simulink library "se2a_controller_lib"  (R2018b)
settings: Solver=VariableStepAuto  StartTime=0.0  StopTime=10.0  RelTol=1e-3
undefined symbols (not defined in the file or in its folder): aircraft, DiscIntNeverNeededParam, gla_indi, pitch_rate_controller
libraries: filters_lib x12, ca_lib x2, simulink x1
settings Model: Creator=Ybeyer  LastModifiedBy=yannic
settings SFSimCC: SimUseLocalCustomCode=off
settings RTWCC: RTWUseLocalCustomCode=off
settings CodeAppCC: StateflowObjectComments=on

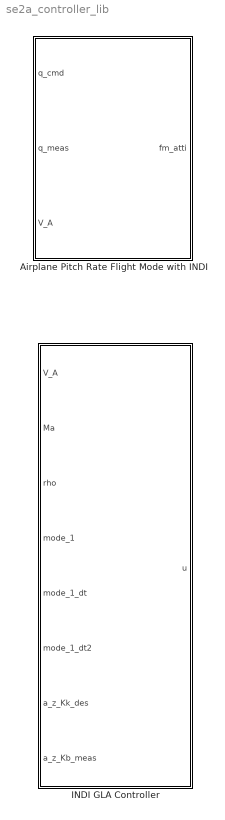
== system se2a_controller_lib ==
  Airplane Pitch Rate Flight Mode with INDI : Subsystem  mask{fm=pitch_rate_controller}
      mask prompts: fm "Pitch rate controller parameters struct"
      mask DialogControl DescGroupVar Prompt: Airplane Pitch Rate Controller with INDI
  INDI GLA Controller : Subsystem  mask{gla_indi=gla_indi}
      mask prompts: gla_indi "Controller parameters struct"
      mask init:
      | % to be controlled mode numbers (non-tunable parameter)
      | mcidx = gla_indi.mcidx;
      mask DialogControl DescGroupVar Prompt: INDI GLA Controller

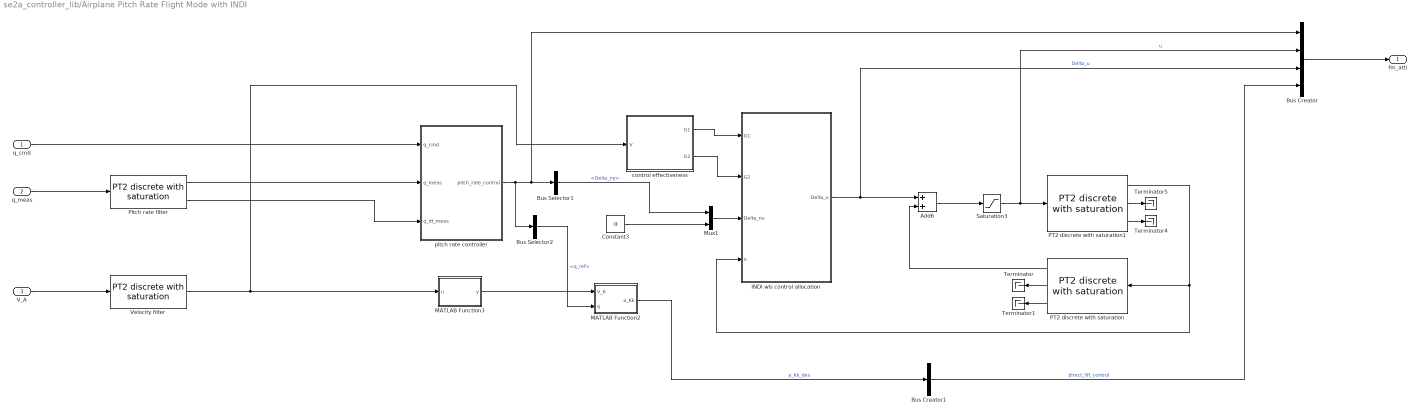
== system se2a_controller_lib/Airplane Pitch Rate Flight Mode with INDI ==
  q_cmd : Inport  SampleTime=fm.sample_time
  q_meas : Inport  Port=2  SampleTime=fm.sample_time
  V_A : Inport  Port=3  SampleTime=fm.sample_time
  Add6 : Sum
  Bus Creator : BusCreator  Inputs=4
  Bus Creator1 : BusCreator  Inputs=1
  Bus Selector1 : BusSelector  OutputSignals=pseudo_control.Delta_ny
  Bus Selector2 : BusSelector  OutputSignals=reference.q_ref
  Constant3 : Constant  Value=0
  INDI wls control allocation : Subsystem  mask{ca=fm.ca, is_Delta_W_v_check=off, is_W_check=off, is_iter_check=off}
      mask prompts: ca "control allocation parameters struct"; is_Delta_W_v_check "enable online adjustment of diag W_v"; is_W_check "enable output "optimal active set" W"; is_iter_check "enable output "number of iterations" iter"
      mask init:
      | caIndiWlsHlcBlockInit(is_Delta_W_v_check,is_W_check,is_iter_check)
      mask DialogControl DescGroupVar Prompt: INDI high level control allocation
      mask DialogControl DescTextVar Prompt: It wraps the INDI control allocation block and adds some high level usability features.
      mask DialogControl Control2 Prompt: This block makes manual throttle control possible. Moreover, it not only considers the control effectiveness G1 but also the effectiveness of the control input derivative G2 [1].
      mask DialogControl Control3 Prompt: [1] Smeur, E. J., Chu, Q., & de Croon, G. C. (2016). Adaptive incremental nonlinear dynamic inversion for attitude control of micro air vehicles. Journal of Guidance, Control, and Dynamics, 39(3), 450-461.
      mask DialogControl Control4 Prompt: To load a control allocation parameters struct, see controlAllocationWlsLoadParams
  MATLAB Function2 : MATLAB Function  TreatAsAtomicUnit=on
  MATLAB Function3 : MATLAB Function  TreatAsAtomicUnit=on
  Mux1 : Mux  Inputs=2
  PT2 discrete with saturation : filters_lib/PT2 discrete with saturation  param_src=internal  omega=fm.sflt.omega  d=fm.sflt.D  x_dt2_max=inf  x_dt2_min=-inf  x_dt_max=inf  x_dt_min=-inf  x_max=inf  x_min=-inf  y_0_src=internal  x_init=0  y_dt_0_src=internal  x_dt_init=0  is_y_dt_checked=on  is_y_dt2_checked=on
      settings: SourceProductName=LADAC
  PT2 discrete with saturation1 : filters_lib/PT2 discrete with saturation  param_src=internal  omega=fm.servo.omega  d=fm.servo.D  x_dt2_max=inf  x_dt2_min=-inf  x_dt_max=inf  x_dt_min=-inf  x_max=inf  x_min=-inf  y_0_src=internal  x_init=0  y_dt_0_src=internal  x_dt_init=0  is_y_dt_checked=on  is_y_dt2_checked=on
      settings: SourceProductName=LADAC
  Pitch rate filter : filters_lib/PT2 discrete with saturation  param_src=internal  omega=fm.sflt.omega  d=fm.sflt.D  x_dt2_max=inf  x_dt2_min=-inf  x_dt_max=inf  x_dt_min=-inf  x_max=inf  x_min=-inf  y_0_src=internal  x_init=0  y_dt_0_src=internal  x_dt_init=0  is_y_dt_checked=on  is_y_dt2_checked=off
      settings: SourceProductName=LADAC
  Saturation3 : Saturate  UpperLimit=fm.ca.u_max  LowerLimit=fm.ca.u_min
  Terminator{,1,4..5} (4 alike) : Terminator
  Velocity filter : filters_lib/PT2 discrete with saturation  param_src=internal  omega=fm.sflt.omega  d=fm.sflt.D  x_dt2_max=inf  x_dt2_min=-inf  x_dt_max=inf  x_dt_min=-inf  x_max=inf  x_min=-inf  y_0_src=internal  x_init=0  y_dt_0_src=internal  x_dt_init=0  is_y_dt_checked=off  is_y_dt2_checked=off
      settings: SourceProductName=LADAC
  control effectiveness : Subsystem
  pitch rate controller : Subsystem
  fm_atti : Outport  SampleTime=fm.sample_time
  wires:
  Constant3/1 -> Mux1/2
  Mux1/1 -> INDI wls control allocation/3(Delta_nu)
  Bus Selector2/1 -> MATLAB Function2/2(q)  "<q_ref>"
  MATLAB Function2/1(a_Kk) -> Bus Creator1/1  "a_Kk_des"
  MATLAB Function3/1(y) -> MATLAB Function2/1(V_K)
  Bus Creator1/1 -> Bus Creator/4  "direct_lift_control"
  Velocity filter/1 -> control effectiveness/1(V), MATLAB Function3/1(u)
  pitch rate controller/1(pitch_rate_control) -> Bus Selector1/1, Bus Creator/1, Bus Selector2/1
  Pitch rate filter/1 -> pitch rate controller/2(q_meas)
  q_cmd/1 -> pitch rate controller/1(q_cmd)
  Saturation3/1 -> Bus Creator/2, PT2 discrete with saturation1/1  "u"
  Bus Selector1/1 -> Mux1/1  "<Delta_ny>"
  PT2 discrete with saturation1/1 -> PT2 discrete with saturation/1, INDI wls control allocation/4(u)
  control effectiveness/2(G2) -> INDI wls control allocation/2(G2)
  Add6/1 -> Saturation3/1
  control effectiveness/1(G1) -> INDI wls control allocation/1(G1)
  INDI wls control allocation/1(Delta_u) -> Add6/1, Bus Creator/3  "Delta_u"
  PT2 discrete with saturation/2 -> Terminator/1
  PT2 discrete with saturation/3 -> Terminator1/1
  Bus Creator/1 -> fm_atti/1
  PT2 discrete with saturation/1 -> Add6/2
  PT2 discrete with saturation1/3 -> Terminator4/1
  PT2 discrete with saturation1/2 -> Terminator5/1
  q_meas/1 -> Pitch rate filter/1
  Pitch rate filter/2 -> pitch rate controller/3(q_dt_meas)
  V_A/1 -> Velocity filter/1

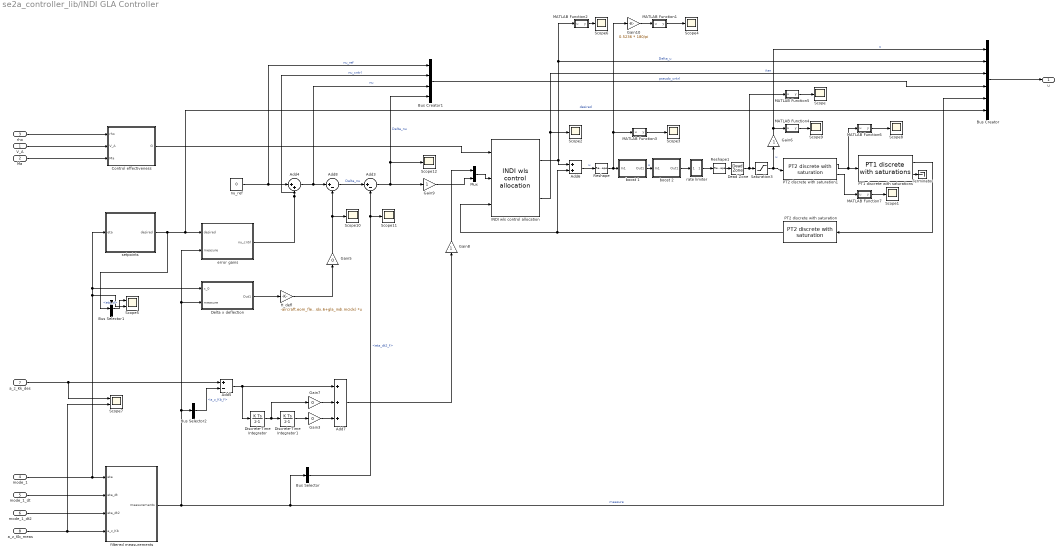
== system se2a_controller_lib/INDI GLA Controller ==
  V_A : Inport  SampleTime=gla_indi.ts
  Ma : Inport  Port=2  SampleTime=gla_indi.ts
  rho : Inport  Port=3  SampleTime=gla_indi.ts
  mode_1 : Inport  Port=4  SampleTime=gla_indi.ts
  mode_1_dt : Inport  Port=5  SampleTime=gla_indi.ts
  mode_1_dt2 : Inport  Port=6  SampleTime=gla_indi.ts
  a_z_Kk_des : Inport  Port=7  SampleTime=gla_indi.ts
  a_z_Kb_meas : Inport  Port=8  SampleTime=gla_indi.ts
  Add3 : Sum  Inputs=|+-
  Add4 : Sum  Inputs=|++
  Add5 : Sum  Inputs=+-
  Add6 : Sum
  Add7 : Sum  Inputs=+++
  Add8 : Sum  Inputs=|+-
  Bus Creator : BusCreator  Inputs=6
  Bus Creator1 : BusCreator  Inputs=4
  Bus Selector : BusSelector  OutputSignals=eta_dt2_f
  Bus Selector1 : BusSelector  OutputSignals=eta_d
  Bus Selector2 : BusSelector  OutputSignals=a_z_Kb_f
  Control effectiveness : Subsystem  mask{cel=gla_indi.ce}
      mask prompts: cel "Control effectiveness parameters struct"
      mask DialogControl DescGroupVar Prompt: Control effectiveness of LADs
  Dead Zone : DeadZone  LowerValue=-gla_indi.udead  UpperValue=gla_indi.udead  SaturateOnIntegerOverflow=on
  Delta x deflection : Subsystem
  Discrete-Time Integrator : DiscreteIntegrator  SampleTime=-1  ICPrevOutput=DiscIntNeverNeededParam  ICPrevScaledInput=DiscIntNeverNeededParam
  Discrete-Time Integrator1 : DiscreteIntegrator  SampleTime=-1  ICPrevOutput=DiscIntNeverNeededParam  ICPrevScaledInput=DiscIntNeverNeededParam
  Gain10 : Gain  Gain=0.5236 * 180/pi
  Gain3 : Gain  Gain=0
  Gain5 : Gain  Gain=0
  Gain6 : Gain
  Gain7 : Gain  Gain=0
  Gain8 : Gain
  Gain9 : Gain
  H_defl : Gain  Gain=-aircraft.eom_flexible.structure_red.M_inv(6+gla_indi.mcidx,6+gla_indi.mcidx)*aircraft.eom_flexible.structure_red.K(6+gla_indi.mcidx,6+gla_indi.mcidx)  Multiplication=Matrix(K*u)
  INDI wls control allocation : ca_lib/INDI wls control allocation  ca=gla_indi.ca  is_Delta_u_d_checked=off  is_Delta_gamma_checked=off  is_Delta_W_v_checked=off  is_Delta_u_max_checked=off  is_W_checked=off  is_iter_checked=on
      settings: SourceProductName=LADAC
  MATLAB Function1 : MATLAB Function  TreatAsAtomicUnit=on
  MATLAB Function2 : MATLAB Function  TreatAsAtomicUnit=on
  MATLAB Function3 : MATLAB Function  TreatAsAtomicUnit=on
  MATLAB Function4 : MATLAB Function  TreatAsAtomicUnit=on
  MATLAB Function5 : MATLAB Function  TreatAsAtomicUnit=on
  MATLAB Function6 : MATLAB Function  TreatAsAtomicUnit=on
  MATLAB Function7 : MATLAB Function  TreatAsAtomicUnit=on
  Mux : Mux  Inputs=2
  PT1 discrete with saturations : filters_lib/PT1 discrete with saturations  T=gla_indi.atc  x_max=inf  x_min=-inf  x_dt_max=inf  x_dt_min=-inf  x_init=0
      settings: SourceProductName=LADAC
  PT2 discrete with saturation : filters_lib/PT2 discrete with saturation  param_src=internal  omega=gla_indi.sflt.omega  d=gla_indi.sflt.d  x_dt2_max=inf  x_dt2_min=-inf  x_dt_max=inf  x_dt_min=-inf  x_max=inf  x_min=-inf  y_0_src=internal  x_init=0  y_dt_0_src=internal  x_dt_init=0  is_y_dt_checked=off  is_y_dt2_checked=off
      settings: SourceProductName=LADAC
  PT2 discrete with saturation1 : filters_lib/PT2 discrete with saturation  param_src=internal  omega=2/gla_indi.dtc  d=1  x_dt2_max=inf  x_dt2_min=-inf  x_dt_max=aircraft.actuators.LAD.defl_rate_max/aircraft.actuators.LAD.defl_max  x_dt_min=aircraft.actuators.LAD.defl_rate_min/aircraft.actuators.LAD.defl_max  x_max=inf  x_min=-inf  y_0_src=internal  x_init=0  y_dt_0_src=internal  x_dt_init=0  is_y_dt_checked=on  is_y_dt2_checked=off
      settings: SourceProductName=LADAC
  Reshape : Reshape  OutputDimensionality=Row vector (2-D)
  Reshape1 : Reshape
  Saturation3 : Saturate  UpperLimit=gla_indi.ca.u_max  LowerLimit=gla_indi.ca.u_min
  Scope{,1..4,6,8..12} (11 alike) : Scope
  Scope5 : Scope  NumInputPorts=2
  Scope7 : Scope  NumInputPorts=2
  Terminator : Terminator
  boost 1 : Subsystem
  boost 2 : Subsystem
  error gains : Subsystem
  filtered measurements : Subsystem
  nu_ref : Constant  Value=0
  rate limiter : Subsystem
  setpoints : Subsystem
  u : Outport
  wires:
  Add4/1 -> Bus Creator1/3, Add8/1  "nu"
  Add8/1 -> Add3/1  "Delta_nu"
  nu_ref/1 -> Add4/1, Bus Creator1/1  "nu_ref"
  filtered measurements/1(measurements) -> Bus Creator/5, Bus Selector/1, Bus Selector2/1, error gains/2(measure), Delta x deflection/2(measure)  "measure"
  INDI wls control allocation/1 -> Add6/1, MATLAB Function2/1(u), Bus Creator/2  "Delta_u"
  Saturation3/1 -> PT2 discrete with saturation1/1, Gain6/1  "u"
  PT1 discrete with saturations/1 -> PT2 discrete with saturation/1
  INDI wls control allocation/2 -> Bus Creator/3, Scope2/1  "iter"
  Dead Zone/1 -> MATLAB Function5/1(u), Saturation3/1
  mode_1_dt/1 -> filtered measurements/2(eta_dt)
  mode_1_dt2/1 -> filtered measurements/3(eta_dt2)
  Bus Creator/1 -> u/1
  error gains/1(nu_cntrl) -> Bus Creator1/2, Add4/2  "nu_cntrl"
  setpoints/1(desired) -> Bus Selector1/1, error gains/1(desired), Bus Creator/6  "desired"
  Bus Creator1/1 -> Bus Creator/4  "pseudo_cntrl"
  Bus Selector/1 -> Add3/2, Scope11/1  "<eta_dt2_f>"
  Control effectiveness/1(G) -> INDI wls control allocation/1
  rho/1 -> Control effectiveness/1(rho)
  V_A/1 -> Control effectiveness/2(V_A)
  Ma/1 -> Control effectiveness/3(Ma)
  H_defl/1 -> Gain5/1
  Gain5/1 -> Add8/2, Scope10/1
  Gain6/1 -> MATLAB Function4/1(u), Bus Creator/1  "u"
  Reshape1/1 -> Dead Zone/1
  Add6/1 -> Reshape/1  "u"
  Reshape/1 -> Gain10/1, MATLAB Function3/1(u), boost 1/1(In1)
  a_z_Kk_des/1 -> Add5/1, Scope7/1
  a_z_Kb_meas/1 -> Scope7/2, filtered measurements/4(a_z_Kb)
  Mux/1 -> INDI wls control allocation/2
  Add5/1 -> Discrete-Time Integrator/1, Add7/1
  Gain8/1 -> Mux/1
  Gain9/1 -> Mux/2
  PT2 discrete with saturation1/1 -> MATLAB Function6/1(u), PT1 discrete with saturations/1
  PT1 discrete with saturations/2 -> Terminator/1
  boost 1/1(Out1) -> boost 2/1(In1)  "u"
  PT2 discrete with saturation/1 -> Add6/2, INDI wls control allocation/3
  Discrete-Time Integrator/1 -> Gain7/1, Discrete-Time Integrator1/1
  Discrete-Time Integrator1/1 -> Gain3/1
  Add7/1 -> Gain8/1
  Gain3/1 -> Add7/3
  Gain7/1 -> Add7/2
  PT2 discrete with saturation1/2 -> MATLAB Function7/1(u)
  Gain10/1 -> MATLAB Function1/1(u)
  MATLAB Function1/1(y) -> Scope4/1
  MATLAB Function2/1(y) -> Scope6/1
  MATLAB Function3/1(y) -> Scope3/1
  MATLAB Function4/1(y) -> Scope9/1
  MATLAB Function5/1(y) -> Scope/1
  MATLAB Function6/1(y) -> Scope8/1
  MATLAB Function7/1(y) -> Scope1/1
  boost 2/1(Out1) -> rate limiter/1(In1)
  rate limiter/1(Out1) -> Reshape1/1
  Add3/1 -> Gain9/1, Bus Creator1/4, Scope12/1  "Delta_nu"
  Delta x deflection/1(Out1) -> H_defl/1
  Bus Selector1/1 -> Scope5/1  "<eta_d>"
  mode_1/1 -> filtered measurements/1(eta), setpoints/1(eta), Delta x deflection/1(x_0), Scope5/2
  Bus Selector2/1 -> Add5/2  "<a_z_Kb_f>"

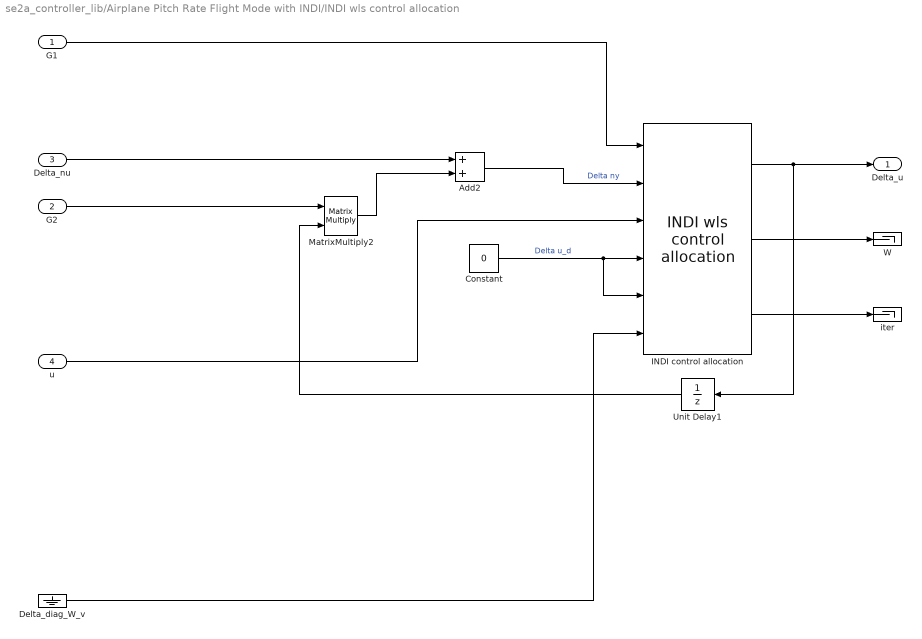
== system se2a_controller_lib/Airplane Pitch Rate Flight Mode with INDI/INDI wls control allocation ==
  G1 : Inport
  G2 : Inport  Port=2
  Delta_nu : Inport  Port=3
  u : Inport  Port=4
  Add2 : Sum
  Constant : Constant  Value=0
  Delta_diag_W_v : Ground
  INDI control allocation : ca_lib/INDI wls control allocation  ca=ca  is_Delta_u_d_checked=on  is_Delta_gamma_checked=on  is_Delta_W_v_checked=on  is_Delta_u_max_checked=off  is_W_checked=on  is_iter_checked=on
      settings: SourceProductName=LADAC
  MatrixMultiply2 : Product  Multiplication=Matrix(*)
  Unit Delay1 : UnitDelay  SampleTime=-1
  W : Terminator
  iter : Terminator
  Delta_u : Outport
  wires:
  G2/1 -> MatrixMultiply2/1
  MatrixMultiply2/1 -> Add2/2
  G1/1 -> INDI control allocation/1
  Add2/1 -> INDI control allocation/2  "Delta ny"
  u/1 -> INDI control allocation/3
  INDI control allocation/1 -> Unit Delay1/1, Delta_u/1
  Delta_nu/1 -> Add2/1
  Unit Delay1/1 -> MatrixMultiply2/2
  Constant/1 -> INDI control allocation/4, INDI control allocation/5  "Delta u_d"
  Delta_diag_W_v/1 -> INDI control allocation/6
  INDI control allocation/3 -> iter/1
  INDI control allocation/2 -> W/1

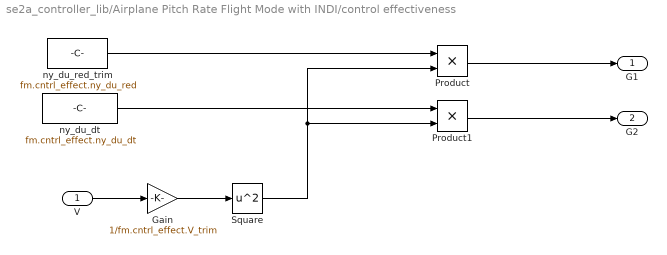
== system se2a_controller_lib/Airplane Pitch Rate Flight Mode with INDI/control effectiveness ==
  V : Inport
  Gain : Gain  Gain=1/fm.cntrl_effect.V_trim
  Product : Product
  Product1 : Product
  Square : Math  Operator=square  SaturateOnIntegerOverflow=on
  ny_du_dt : Constant  Value=fm.cntrl_effect.ny_du_dt
  ny_du_red_trim : Constant  Value=fm.cntrl_effect.ny_du_red
  G1 : Outport
  G2 : Outport  Port=2
  wires:
  ny_du_dt/1 -> Product1/1
  ny_du_red_trim/1 -> Product/1
  V/1 -> Gain/1
  Gain/1 -> Square/1
  Product/1 -> G1/1
  Square/1 -> Product1/2, Product/2
  Product1/1 -> G2/1

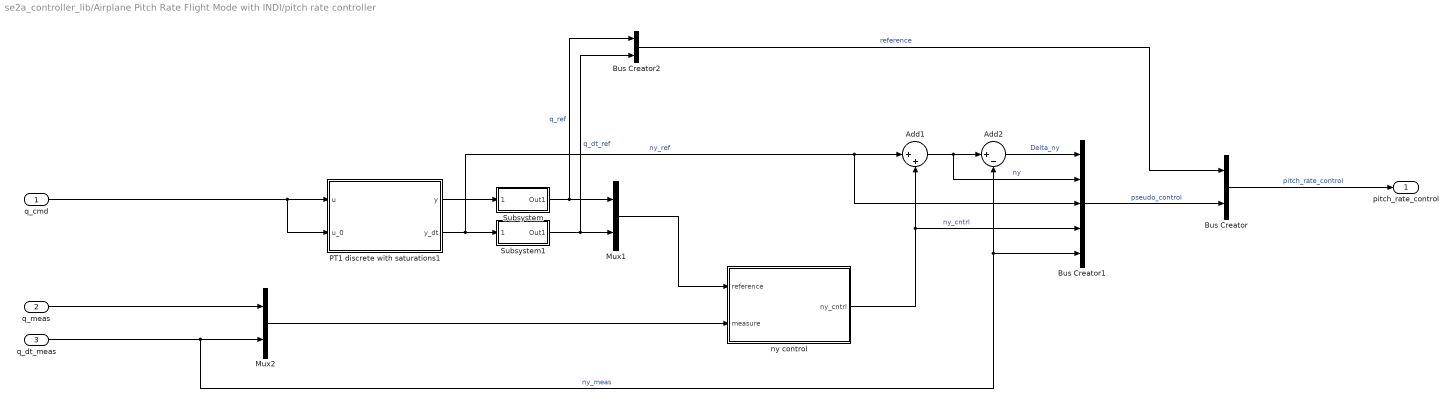
== system se2a_controller_lib/Airplane Pitch Rate Flight Mode with INDI/pitch rate controller ==
  q_cmd : Inport
  q_meas : Inport  Port=2
  q_dt_meas : Inport  Port=3
  Add1 : Sum  Inputs=|++
  Add2 : Sum  Inputs=|+-
  Bus Creator : BusCreator  Inputs=2
  Bus Creator1 : BusCreator  Inputs=5
  Bus Creator2 : BusCreator  Inputs=2
  Mux1 : Mux  Inputs=2
  Mux2 : Mux  Inputs=2
  PT1 discrete with saturations1 : Subsystem  mask{T=fm.rm.T, x_max=inf, x_min=-inf, x_dt_max=inf, x_dt_min=-inf, x_init=0}
      mask prompts: T "Time constant"; x_max "Maximum output"; x_min "Minimum output"; x_dt_max "Maximum output rate"; x_dt_min "Minimum output rate"; x_init "Initial output"
  Subsystem : Subsystem
  Subsystem1 : Subsystem
  ny control : Subsystem
  pitch_rate_control : Outport
  wires:
  Bus Creator2/1 -> Bus Creator/1  "reference"
  Mux2/1 -> ny control/2(measure)
  ny control/1(ny_cntrl) -> Add1/2, Bus Creator1/4  "ny_cntrl"
  q_dt_meas/1 -> Mux2/2, Bus Creator1/5, Add2/2  "ny_meas"
  q_meas/1 -> Mux2/1
  Subsystem1/1(Out1) -> Mux1/2, Bus Creator2/2  "q_dt_ref"
  q_cmd/1 -> PT1 discrete with saturations1/1(u), PT1 discrete with saturations1/2("u_0 ")
  Subsystem/1(Out1) -> Mux1/1, Bus Creator2/1  "q_ref"
  PT1 discrete with saturations1/2(y_dt) -> Add1/1, Bus Creator1/3, Subsystem1/1(<x_ref>)  "ny_ref"
  Add2/1 -> Bus Creator1/1  "Delta_ny"
  Bus Creator/1 -> pitch_rate_control/1  "pitch_rate_control"
  PT1 discrete with saturations1/1(y) -> Subsystem/1(<x_ref>)
  Bus Creator1/1 -> Bus Creator/2  "pseudo_control"
  Add1/1 -> Bus Creator1/2, Add2/1  "ny"
  Mux1/1 -> ny control/1(reference)

== system se2a_controller_lib/INDI GLA Controller/Control effectiveness ==
  rho : Inport
  V_A : Inport  Port=2
  Ma : Inport  Port=3
  Control effectiveness : MATLAB Function  TreatAsAtomicUnit=on
  G : Outport
  wires:
  Ma/1 -> Control effectiveness/3(Ma)
  rho/1 -> Control effectiveness/1(rho)
  Control effectiveness/1(G) -> G/1
  V_A/1 -> Control effectiveness/2(V_A)

== system se2a_controller_lib/INDI GLA Controller/Delta x deflection ==
  x_0 : Inport
  measure : Inport  Port=2
  Add2 : Sum  Inputs=+-
  Bus Selector1 : BusSelector  OutputSignals=eta_f
  Out1 : Outport
  wires:
  x_0/1 -> Add2/1  "eta_dt_f"
  measure/1 -> Bus Selector1/1
  Bus Selector1/1 -> Add2/2  "<eta_f>"
  Add2/1 -> Out1/1

== system se2a_controller_lib/INDI GLA Controller/boost 1 ==
  In1 : Inport
  boost 11 : Subsystem
  boost 12 : Subsystem
  Out1 : Outport
  wires:
  boost 11/1(Out1) -> boost 12/1(In1)
  boost 12/1(Out1) -> Out1/1
  In1/1 -> boost 11/1(In1)

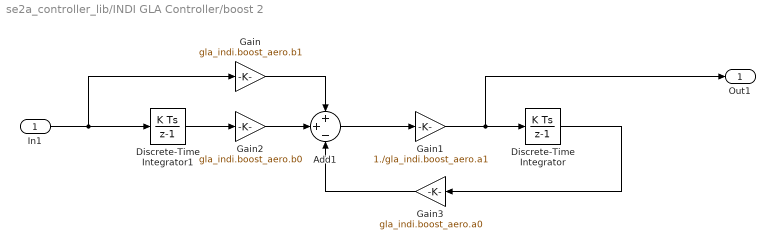
== system se2a_controller_lib/INDI GLA Controller/boost 2 ==
  In1 : Inport
  Add1 : Sum  Inputs=++-
  Discrete-Time Integrator : DiscreteIntegrator  SampleTime=-1  ICPrevOutput=DiscIntNeverNeededParam  ICPrevScaledInput=DiscIntNeverNeededParam
  Discrete-Time Integrator1 : DiscreteIntegrator  SampleTime=-1  ICPrevOutput=DiscIntNeverNeededParam  ICPrevScaledInput=DiscIntNeverNeededParam
  Gain : Gain  Gain=gla_indi.boost_aero.b1
  Gain1 : Gain  Gain=1./gla_indi.boost_aero.a1
  Gain2 : Gain  Gain=gla_indi.boost_aero.b0
  Gain3 : Gain  Gain=gla_indi.boost_aero.a0
  Out1 : Outport
  wires:
  In1/1 -> Gain/1, Discrete-Time Integrator1/1
  Gain/1 -> Add1/1
  Add1/1 -> Gain1/1
  Gain2/1 -> Add1/2
  Discrete-Time Integrator/1 -> Gain3/1
  Gain3/1 -> Add1/3
  Discrete-Time Integrator1/1 -> Gain2/1
  Gain1/1 -> Out1/1, Discrete-Time Integrator/1

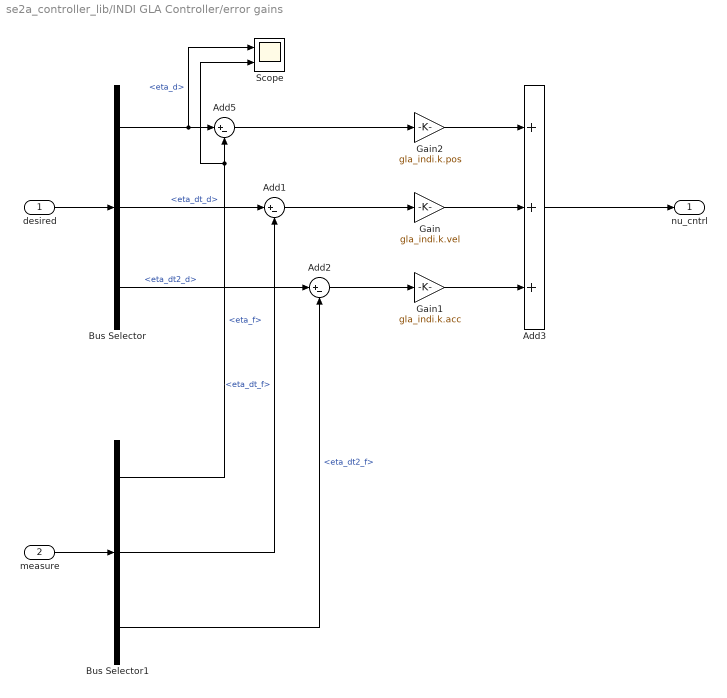
== system se2a_controller_lib/INDI GLA Controller/error gains ==
  desired : Inport
  measure : Inport  Port=2
  Add1 : Sum  Inputs=|+-
  Add2 : Sum  Inputs=|+-
  Add3 : Sum  Inputs=+++
  Add5 : Sum  Inputs=|+-
  Bus Selector : BusSelector  OutputSignals=eta_d,eta_dt_d,eta_dt2_d
  Bus Selector1 : BusSelector  OutputSignals=eta_f,eta_dt_f,eta_dt2_f
  Gain : Gain  Gain=gla_indi.k.vel
  Gain1 : Gain  Gain=gla_indi.k.acc
  Gain2 : Gain  Gain=gla_indi.k.pos
  Scope : Scope  NumInputPorts=2
  nu_cntrl : Outport
  wires:
  Add2/1 -> Gain1/1
  Add1/1 -> Gain/1
  Gain/1 -> Add3/2
  Bus Selector/1 -> Scope/1, Add5/1  "<eta_d>"
  Gain2/1 -> Add3/1
  Bus Selector/2 -> Add1/1  "<eta_dt_d>"
  Bus Selector1/2 -> Add1/2  "<eta_dt_f>"
  Bus Selector1/3 -> Add2/2  "<eta_dt2_f>"
  Add5/1 -> Gain2/1
  Bus Selector/3 -> Add2/1  "<eta_dt2_d>"
  Gain1/1 -> Add3/3
  Add3/1 -> nu_cntrl/1
  desired/1 -> Bus Selector/1
  measure/1 -> Bus Selector1/1
  Bus Selector1/1 -> Scope/2, Add5/2  "<eta_f>"

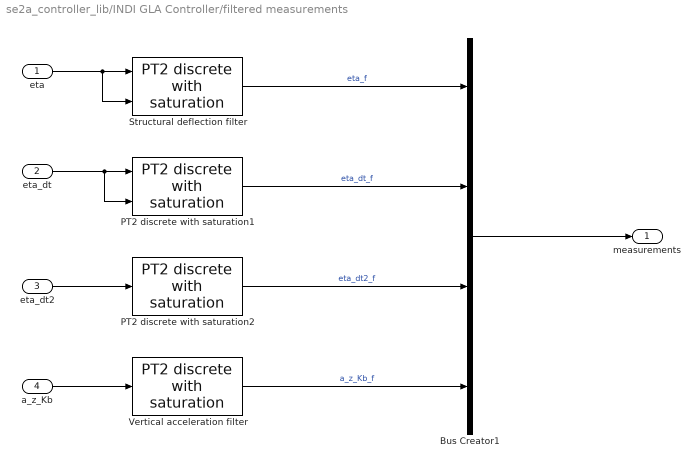
== system se2a_controller_lib/INDI GLA Controller/filtered measurements ==
  eta : Inport
  eta_dt : Inport  Port=2
  eta_dt2 : Inport  Port=3
  a_z_Kb : Inport  Port=4
  Bus Creator1 : BusCreator  Inputs=4
  PT2 discrete with saturation1 : filters_lib/PT2 discrete with saturation  param_src=internal  omega=gla_indi.sflt.omega  d=gla_indi.sflt.d  x_dt2_max=inf  x_dt2_min=-inf  x_dt_max=inf  x_dt_min=-inf  x_max=inf  x_min=-inf  y_0_src=external  x_init=0  y_dt_0_src=internal  x_dt_init=0  is_y_dt_checked=off  is_y_dt2_checked=off
      settings: SourceProductName=LADAC
  PT2 discrete with saturation2 : filters_lib/PT2 discrete with saturation  param_src=internal  omega=gla_indi.sflt.omega  d=gla_indi.sflt.d  x_dt2_max=inf  x_dt2_min=-inf  x_dt_max=inf  x_dt_min=-inf  x_max=inf  x_min=-inf  y_0_src=internal  x_init=0  y_dt_0_src=internal  x_dt_init=0  is_y_dt_checked=off  is_y_dt2_checked=off
      settings: SourceProductName=LADAC
  Structural deflection filter : filters_lib/PT2 discrete with saturation  param_src=internal  omega=gla_indi.sflt.omega  d=gla_indi.sflt.d  x_dt2_max=inf  x_dt2_min=-inf  x_dt_max=inf  x_dt_min=-inf  x_max=inf  x_min=-inf  y_0_src=external  x_init=0  y_dt_0_src=internal  x_dt_init=0  is_y_dt_checked=off  is_y_dt2_checked=off
      settings: SourceProductName=LADAC
  Vertical acceleration filter : filters_lib/PT2 discrete with saturation  param_src=internal  omega=gla_indi.sflt.omega  d=gla_indi.sflt.d  x_dt2_max=inf  x_dt2_min=-inf  x_dt_max=inf  x_dt_min=-inf  x_max=inf  x_min=-inf  y_0_src=internal  x_init=0  y_dt_0_src=internal  x_dt_init=0  is_y_dt_checked=off  is_y_dt2_checked=off
      settings: SourceProductName=LADAC
  measurements : Outport
  wires:
  eta/1 -> Structural deflection filter/2, Structural deflection filter/1
  Structural deflection filter/1 -> Bus Creator1/1  "eta_f"
  PT2 discrete with saturation1/1 -> Bus Creator1/2  "eta_dt_f"
  PT2 discrete with saturation2/1 -> Bus Creator1/3  "eta_dt2_f"
  eta_dt/1 -> PT2 discrete with saturation1/2, PT2 discrete with saturation1/1
  eta_dt2/1 -> PT2 discrete with saturation2/1
  Bus Creator1/1 -> measurements/1
  a_z_Kb/1 -> Vertical acceleration filter/1
  Vertical acceleration filter/1 -> Bus Creator1/4  "a_z_Kb_f"

== system se2a_controller_lib/INDI GLA Controller/rate limiter ==
  In1 : Inport
  Constant : Constant  Value=aircraft.actuators.LAD.defl_rate_max/aircraft.actuators.LAD.defl_max
  Constant1 : Constant  Value=aircraft.actuators.LAD.defl_rate_min/aircraft.actuators.LAD.defl_max
  Gain : Gain  Gain=300
  Gain1 : Gain  Gain=300
  Rate Limiter Dynamic : simulink/Discontinuities/Rate Limiter Dynamic
      settings: SourceProductName=Simulink
  Out1 : Outport
  wires:
  In1/1 -> Rate Limiter Dynamic/2
  Rate Limiter Dynamic/1 -> Out1/1
  Constant/1 -> Gain/1
  Constant1/1 -> Gain1/1
  Gain/1 -> Rate Limiter Dynamic/1
  Gain1/1 -> Rate Limiter Dynamic/3

== system se2a_controller_lib/INDI GLA Controller/setpoints ==
  eta : Inport
  Bus Creator : BusCreator  Inputs=3
  Constant2 : Constant  Value=0
  Constant3 : Constant  Value=0
  Gain : Gain
  PT2 discrete with saturation : filters_lib/PT2 discrete with saturation  param_src=internal  omega=gla_indi.ref.omega  d=gla_indi.ref.d  x_dt2_max=inf  x_dt2_min=-inf  x_dt_max=inf  x_dt_min=-inf  x_max=inf  x_min=-inf  y_0_src=internal  x_init=0  y_dt_0_src=internal  x_dt_init=0  is_y_dt_checked=off  is_y_dt2_checked=off
      settings: SourceProductName=LADAC
  desired : Outport
  wires:
  eta/1 -> PT2 discrete with saturation/1
  Constant3/1 -> Bus Creator/3  "eta_dt2_d"
  Constant2/1 -> Bus Creator/2  "eta_dt_d"
  PT2 discrete with saturation/1 -> Gain/1
  Bus Creator/1 -> desired/1
  Gain/1 -> Bus Creator/1  "eta_d"

== system se2a_controller_lib/Airplane Pitch Rate Flight Mode with INDI/pitch rate controller/PT1 discrete with saturations1 ==
  u : Inport
  "u_0 " : Inport  Port=2
  1/T : Gain  Gain=1./T
  Discrete-Time Integrator : DiscreteIntegrator  InitialConditionSource=external  InitialCondition=x_init  SampleTime=-1  LimitOutput=on  UpperSaturationLimit=x_max  LowerSaturationLimit=x_min  ICPrevOutput=DiscIntNeverNeededParam  ICPrevScaledInput=DiscIntNeverNeededParam
  Saturation : Saturate  UpperLimit=x_dt_max  LowerLimit=x_dt_min
  Sum2 : Sum  Inputs=|+-
  y : Outport
  y_dt : Outport  Port=2
  wires:
  "u_0 "/1 -> Discrete-Time Integrator/2
  1/T/1 -> Saturation/1
  u/1 -> Sum2/1
  Sum2/1 -> 1/T/1
  Discrete-Time Integrator/1 -> Sum2/2, y/1  "y"
  Saturation/1 -> y_dt/1, Discrete-Time Integrator/1  "y_dt"

== system se2a_controller_lib/Airplane Pitch Rate Flight Mode with INDI/pitch rate controller/Subsystem ==
  <x_ref> : Inport
  PT2 discrete with saturation : Subsystem  mask{omega=2./(2/fm.sflt.omega + 2/fm.servo.omega), d=1, x_dt2_max=inf, x_dt2_min=-inf, x_dt_max=inf, x_dt_min=-inf, x_max=inf, x_min=-inf, x_init=0, x_dt_init=0}
      mask prompts: omega "Natural frequency"; d "Damping ratio"; x_dt2_max "Maximum acceleration"; x_dt2_min "Minimum acceleration"; x_dt_max "Maximum rate"; x_dt_min "Minimum rate"; x_max "Maximum position"; x_min "Minimum position"; x_init "Initial position"; x_dt_init "Initial rate"
  Terminator : Terminator
  Terminator1 : Terminator
  Out1 : Outport
  wires:
  PT2 discrete with saturation/2(y_dt) -> Terminator/1
  PT2 discrete with saturation/3(y_dt2) -> Terminator1/1
  PT2 discrete with saturation/1(y) -> Out1/1
  <x_ref>/1 -> PT2 discrete with saturation/2(u_0), PT2 discrete with saturation/1(u)

== system se2a_controller_lib/Airplane Pitch Rate Flight Mode with INDI/pitch rate controller/Subsystem1 ==
  <x_ref> : Inport
  PT2 discrete with saturation : Subsystem  mask{omega=2./(2/fm.sflt.omega + 2/fm.servo.omega), d=1, x_dt2_max=inf, x_dt2_min=-inf, x_dt_max=inf, x_dt_min=-inf, x_max=inf, x_min=-inf, x_init=0, x_dt_init=0}
      mask prompts: omega "Natural frequency"; d "Damping ratio"; x_dt2_max "Maximum acceleration"; x_dt2_min "Minimum acceleration"; x_dt_max "Maximum rate"; x_dt_min "Minimum rate"; x_max "Maximum position"; x_min "Minimum position"; x_init "Initial position"; x_dt_init "Initial rate"
  Terminator : Terminator
  Terminator1 : Terminator
  Out1 : Outport
  wires:
  PT2 discrete with saturation/2(y_dt) -> Terminator/1
  PT2 discrete with saturation/3(y_dt2) -> Terminator1/1
  PT2 discrete with saturation/1(y) -> Out1/1
  <x_ref>/1 -> PT2 discrete with saturation/2(u_0), PT2 discrete with saturation/1(u)

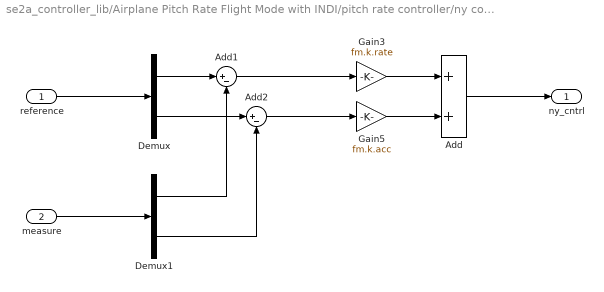
== system se2a_controller_lib/Airplane Pitch Rate Flight Mode with INDI/pitch rate controller/ny control ==
  reference : Inport
  measure : Inport  Port=2
  Add : Sum  Inputs=2
  Add1 : Sum  Inputs=|+-
  Add2 : Sum  Inputs=|+-
  Demux : Demux  Outputs=2
  Demux1 : Demux  Outputs=2
  Gain3 : Gain  Gain=fm.k.rate
  Gain5 : Gain  Gain=fm.k.acc
  ny_cntrl : Outport
  wires:
  Demux1/2 -> Add2/2
  Demux1/1 -> Add1/2
  Add2/1 -> Gain5/1
  Add1/1 -> Gain3/1
  measure/1 -> Demux1/1
  reference/1 -> Demux/1
  Demux/1 -> Add1/1
  Demux/2 -> Add2/1
  Gain5/1 -> Add/2
  Gain3/1 -> Add/1
  Add/1 -> ny_cntrl/1

== system se2a_controller_lib/INDI GLA Controller/boost 1/boost 11 ==
  In1 : Inport
  Add1 : Sum  Inputs=++-
  Discrete-Time Integrator : DiscreteIntegrator  SampleTime=-1  ICPrevOutput=DiscIntNeverNeededParam  ICPrevScaledInput=DiscIntNeverNeededParam
  Discrete-Time Integrator1 : DiscreteIntegrator  SampleTime=-1  ICPrevOutput=DiscIntNeverNeededParam  ICPrevScaledInput=DiscIntNeverNeededParam
  Gain : Gain  Gain=gla_indi.boost_servo.b1
  Gain1 : Gain  Gain=1./gla_indi.boost_servo.a1
  Gain2 : Gain  Gain=gla_indi.boost_servo.b0
  Gain3 : Gain  Gain=gla_indi.boost_servo.a0
  Out1 : Outport
  wires:
  In1/1 -> Gain/1, Discrete-Time Integrator1/1
  Gain/1 -> Add1/1
  Add1/1 -> Gain1/1
  Gain2/1 -> Add1/2
  Discrete-Time Integrator/1 -> Gain3/1
  Gain3/1 -> Add1/3
  Discrete-Time Integrator1/1 -> Gain2/1
  Gain1/1 -> Out1/1, Discrete-Time Integrator/1

== system se2a_controller_lib/INDI GLA Controller/boost 1/boost 12 ==
  In1 : Inport
  Add1 : Sum  Inputs=++-
  Discrete-Time Integrator : DiscreteIntegrator  SampleTime=-1  ICPrevOutput=DiscIntNeverNeededParam  ICPrevScaledInput=DiscIntNeverNeededParam
  Discrete-Time Integrator1 : DiscreteIntegrator  SampleTime=-1  ICPrevOutput=DiscIntNeverNeededParam  ICPrevScaledInput=DiscIntNeverNeededParam
  Gain : Gain  Gain=gla_indi.boost_servo.b1
  Gain1 : Gain  Gain=1./gla_indi.boost_servo.a1
  Gain2 : Gain  Gain=gla_indi.boost_servo.b0
  Gain3 : Gain  Gain=gla_indi.boost_servo.a0
  Out1 : Outport
  wires:
  Gain1/1 -> Discrete-Time Integrator/1, Out1/1
  Discrete-Time Integrator1/1 -> Gain2/1
  Gain3/1 -> Add1/3
  Discrete-Time Integrator/1 -> Gain3/1
  Gain2/1 -> Add1/2
  Add1/1 -> Gain1/1
  Gain/1 -> Add1/1
  In1/1 -> Discrete-Time Integrator1/1, Gain/1

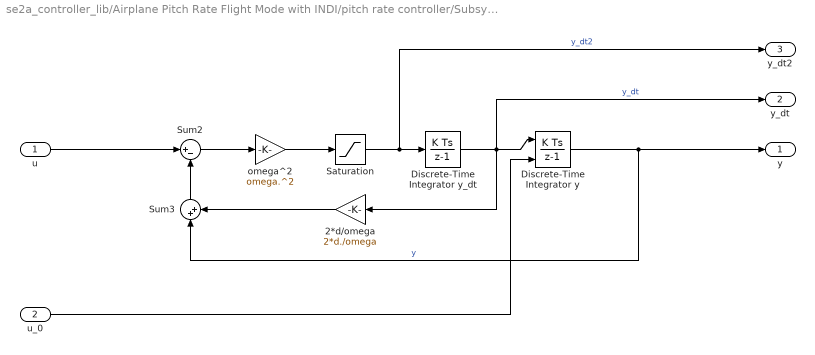
== system se2a_controller_lib/Airplane Pitch Rate Flight Mode with INDI/pitch rate controller/Subsystem/PT2 discrete with saturation ==
  u : Inport
  u_0 : Inport  Port=2
  2*d/omega : Gain  Gain=2*d./omega
  Discrete-Time Integrator y : DiscreteIntegrator  InitialConditionSource=external  InitialCondition=x_init  SampleTime=-1  OutDataTypeStr=Inherit: Inherit via back propagation  LimitOutput=on  UpperSaturationLimit=x_max  LowerSaturationLimit=x_min  ICPrevOutput=DiscIntNeverNeededParam  ICPrevScaledInput=DiscIntNeverNeededParam
  Discrete-Time Integrator y_dt : DiscreteIntegrator  InitialCondition=x_dt_init  SampleTime=-1  OutDataTypeStr=Inherit: Inherit via back propagation  LimitOutput=on  UpperSaturationLimit=x_dt_max  LowerSaturationLimit=x_dt_min  ICPrevOutput=DiscIntNeverNeededParam  ICPrevScaledInput=DiscIntNeverNeededParam
  Saturation : Saturate  UpperLimit=x_dt2_max  LowerLimit=x_dt2_min
  Sum2 : Sum  Inputs=|+-
  Sum3 : Sum  Inputs=|++
  omega^2 : Gain  Gain=omega.^2
  y : Outport
  y_dt : Outport  Port=2
  y_dt2 : Outport  Port=3
  wires:
  Saturation/1 -> y_dt2/1, Discrete-Time Integrator y_dt/1  "y_dt2"
  omega^2/1 -> Saturation/1
  Sum3/1 -> Sum2/2
  u/1 -> Sum2/1
  2*d/omega/1 -> Sum3/2
  Sum2/1 -> omega^2/1
  Discrete-Time Integrator y/1 -> Sum3/1, y/1  "y"
  Discrete-Time Integrator y_dt/1 -> 2*d/omega/1, y_dt/1, Discrete-Time Integrator y/1  "y_dt"
  u_0/1 -> Discrete-Time Integrator y/2

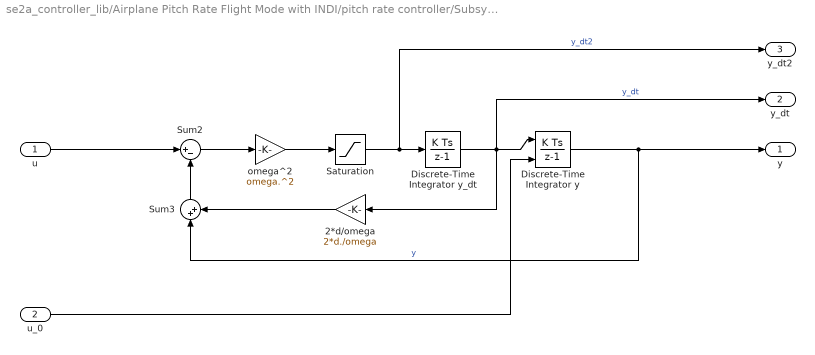
== system se2a_controller_lib/Airplane Pitch Rate Flight Mode with INDI/pitch rate controller/Subsystem1/PT2 discrete with saturation ==
  u : Inport
  u_0 : Inport  Port=2
  2*d/omega : Gain  Gain=2*d./omega
  Discrete-Time Integrator y : DiscreteIntegrator  InitialConditionSource=external  InitialCondition=x_init  SampleTime=-1  OutDataTypeStr=Inherit: Inherit via back propagation  LimitOutput=on  UpperSaturationLimit=x_max  LowerSaturationLimit=x_min  ICPrevOutput=DiscIntNeverNeededParam  ICPrevScaledInput=DiscIntNeverNeededParam
  Discrete-Time Integrator y_dt : DiscreteIntegrator  InitialCondition=x_dt_init  SampleTime=-1  OutDataTypeStr=Inherit: Inherit via back propagation  LimitOutput=on  UpperSaturationLimit=x_dt_max  LowerSaturationLimit=x_dt_min  ICPrevOutput=DiscIntNeverNeededParam  ICPrevScaledInput=DiscIntNeverNeededParam
  Saturation : Saturate  UpperLimit=x_dt2_max  LowerLimit=x_dt2_min
  Sum2 : Sum  Inputs=|+-
  Sum3 : Sum  Inputs=|++
  omega^2 : Gain  Gain=omega.^2
  y : Outport
  y_dt : Outport  Port=2
  y_dt2 : Outport  Port=3
  wires:
  Saturation/1 -> y_dt2/1, Discrete-Time Integrator y_dt/1  "y_dt2"
  omega^2/1 -> Saturation/1
  Sum3/1 -> Sum2/2
  u/1 -> Sum2/1
  2*d/omega/1 -> Sum3/2
  Sum2/1 -> omega^2/1
  Discrete-Time Integrator y/1 -> Sum3/1, y/1  "y"
  Discrete-Time Integrator y_dt/1 -> 2*d/omega/1, y_dt/1, Discrete-Time Integrator y/1  "y_dt"
  u_0/1 -> Discrete-Time Integrator y/2

== matlab function se2a_controller_lib/INDI GLA Controller/Control effectiveness/Control effectiveness ==
  data: G output; rho input; V_A input; Ma input; cel parameter
function G = indiCeLadVar( rho, V_A, Ma,  cel)
G = indiCeLadVar( cel, rho, V_A, Ma );
end

== matlab function se2a_controller_lib/Airplane Pitch Rate Flight Mode with INDI/MATLAB Function2 ==
  data: V_K input; a_Kk output; q input
function a_Kk = fcn(V_K,q)
V_Kk = [V_K;0;0];
Omega_Kk = [0;q;0];
a_Kk = cross(Omega_Kk,V_Kk);
end

== matlab function se2a_controller_lib/INDI GLA Controller/MATLAB Function1 ==
  data: u input; y output
function y  = fcn(u)

y = u(1:19);

== matlab function se2a_controller_lib/INDI GLA Controller/MATLAB Function2 ==
  data: u input; y output
function y  = fcn(u)

y = u(1:19);

== matlab function se2a_controller_lib/Airplane Pitch Rate Flight Mode with INDI/MATLAB Function3 ==
  data: u input; y output
function y = fcn(u)
y=norm(u,2);
end

== matlab function se2a_controller_lib/INDI GLA Controller/MATLAB Function3 ==
  data: u input; y output
function y  = fcn(u)

y = u(1:19);

== matlab function se2a_controller_lib/INDI GLA Controller/MATLAB Function4 ==
  data: u input; y output
function y  = fcn(u)

y = u(1:19);

== matlab function se2a_controller_lib/INDI GLA Controller/MATLAB Function5 ==
  data: u input; y output
function y  = fcn(u)

y = u(1:19);

== matlab function se2a_controller_lib/INDI GLA Controller/MATLAB Function6 ==
  data: u input; y output
function y  = fcn(u)

y = u(1:19);

== matlab function se2a_controller_lib/INDI GLA Controller/MATLAB Function7 ==
  data: u input; y output
function y  = fcn(u)

y = u(1:19);
